simulink model "Model2_Test_Exists"  (R2018b)
settings: Solver=ode8  StartTime=0.0  StopTime=100.0  FixedStep=0.01  RelTol=1e-6
undefined symbols (not defined in the file or in its folder): tollerableriskTest_Exists
settings Model: SimulationMode=accelerator  Creator=claudio.menghi  LastModifiedBy=claudio.menghi
settings SolverCC: MaxConsecutiveZCs=10000  ShapePreserveControl=EnableAll  ZeroCrossControl=EnableAll  ZeroCrossAlgorithm=Adaptive  AutoInsertRateTranBlk=on

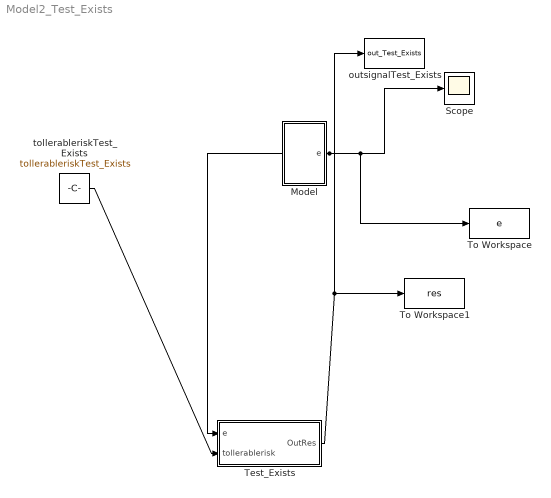
== system Model2_Test_Exists ==
  Model : Subsystem
  Scope : Scope
  Test_Exists : Subsystem
  To Workspace : ToWorkspace  VariableName=e  SaveFormat=Timeseries  SampleTime=-1
  To Workspace1 : ToWorkspace  VariableName=res  SaveFormat=Timeseries  SampleTime=-1
  outsignalTest_Exists : ToWorkspace  VariableName=out_Test_Exists  SaveFormat=Timeseries  SampleTime=-1
      settings: MaxDataPoints=1
  tollerableriskTest_Exists : Constant  Value=tollerableriskTest_Exists
  wires:
  Model/1(e) -> To Workspace/1, Scope/1, Test_Exists/1(e)
  tollerableriskTest_Exists/1 -> Test_Exists/2(tollerablerisk)
  Test_Exists/1(OutRes) -> To Workspace1/1, outsignalTest_Exists/1

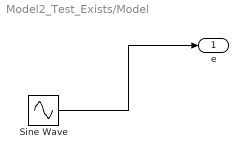
== system Model2_Test_Exists/Model ==
  Sine Wave : Sin  Amplitude=0.5  SampleTime=0
  e : Outport
  wires:
  Sine Wave/1 -> e/1

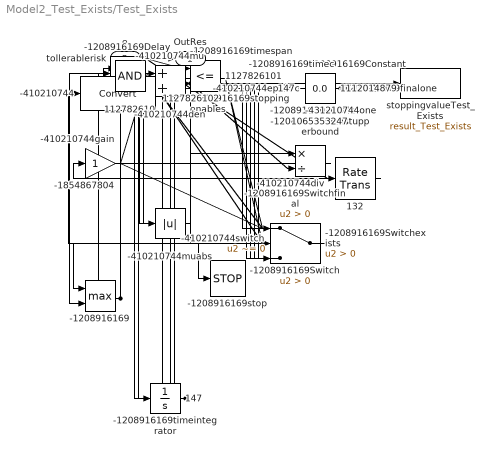
== system Model2_Test_Exists/Test_Exists ==
  e : Inport
  tollerablerisk : Inport  Port=2
  -1208916169 : MinMax  Function=max  Inputs=2
  -1208916169Constant : Constant  Value=-1
  -1208916169Delay : UnitDelay  InitialCondition=-1  SampleTime=-1
  -1208916169Switch : Switch  Criteria=u2 > Threshold
  -1208916169Switchexists : Switch  Criteria=u2 > Threshold
  -1208916169Switchfinal : Switch  Criteria=u2 > Threshold
  -1208916169existupperbound : Constant  Value=50.0
  -1208916169finalone : Constant
  -1208916169finalzero : Constant  Value=0
  -1208916169stop : Stop
  -1208916169stoppingenables : RelationalOperator  OutDataTypeStr=boolean  RndMeth=Simplest
  -1208916169timec : Constant
  -1208916169timeintegrator : Integrator
  -1208916169timespan : RelationalOperator  OutDataTypeStr=boolean  RndMeth=Simplest
  -1854867804 : Gain
  -410210744 : DataTypeConversion
  -410210744den : Sum
  -410210744div : Product  Inputs=*/
  -410210744epsilon : Constant  Value=-0.01
  -410210744gain : Gain
  -410210744mu : Sum  Inputs=+-
  -410210744muabs : Abs
  -410210744one : Constant
  -410210744switch : Switch  Criteria=u2 ~= 0
  1065353247 : Constant  Value=1.0
  1112014879 : Constant  Value=50.0
  112782610 : Logic  AllPortsSameDT=off  OutDataTypeStr=boolean
  1127826101 : RelationalOperator  Operator=<=  OutDataTypeStr=boolean  RndMeth=Simplest
  1127826102 : RelationalOperator  Operator=<=  OutDataTypeStr=boolean  RndMeth=Simplest
  132 : RateTransition
  147 : Integrator
  147c : Constant
  31 : Constant  Value=0.0
  stoppingvalueTest_Exists : ToWorkspace  VariableName=result_Test_Exists  SaveFormat=Timeseries  SampleTime=-1
      settings: MaxDataPoints=1
  OutRes : Outport
  wires:
  147c/1 -> 147/1
  31/1 -> 1127826101/1
  147/1 -> 1127826101/2, 1127826102/1
  1112014879/1 -> 1127826102/2
  1127826101/1 -> 112782610/1
  1127826102/1 -> 112782610/2
  e/1 -> 132/1
  132/1 -> -1854867804/1
  -1854867804/1 -> -410210744mu/1
  1065353247/1 -> -410210744mu/2
  -410210744mu/1 -> -410210744muabs/1, -410210744div/1, -410210744switch/2
  -410210744muabs/1 -> -410210744den/1
  -410210744one/1 -> -410210744den/2
  -410210744den/1 -> -410210744div/2
  -410210744div/1 -> -410210744gain/1
  -410210744gain/1 -> -410210744switch/1
  -410210744epsilon/1 -> -410210744switch/3
  -410210744switch/1 -> -410210744/1
  -1208916169Constant/1 -> -1208916169Switch/3
  112782610/1 -> -1208916169Switch/2
  -410210744/1 -> -1208916169Switch/1
  -1208916169Switch/1 -> -1208916169/1
  -1208916169/1 -> -1208916169Delay/1, OutRes/1, -1208916169timespan/2, stoppingvalueTest_Exists/1
  -1208916169Delay/1 -> -1208916169/2
  tollerablerisk/1 -> -1208916169timespan/1
  -1208916169finalzero/1 -> -1208916169Switchfinal/3, -1208916169Switchexists/3
  -1208916169timec/1 -> -1208916169timeintegrator/1
  -1208916169timeintegrator/1 -> -1208916169stoppingenables/1
  -1208916169existupperbound/1 -> -1208916169stoppingenables/2
  -1208916169stoppingenables/1 -> -1208916169Switchexists/2
  -1208916169timespan/1 -> -1208916169Switchexists/1
  -1208916169finalone/1 -> -1208916169Switchfinal/1
  -1208916169Switchexists/1 -> -1208916169Switchfinal/2
  -1208916169Switchfinal/1 -> -1208916169stop/1
